simulink model "saturn_thermal5"  (R2021a)
settings: Solver=ode23t  StartTime=0.0  StopTime=t_simul  MaxStep=3600  MinStep=1  RelTol=0.1
values from neighbouring files (symbols this model uses):
  Ab = L*l    [Data_ini_thermal_analysis4.m]    (also in Data_ini_thermal_analysis5.m)
  Ant_Heater_MaxPower = 250    [Data_ini_thermal_analysis5.m]
  As = l*l    [Data_ini_thermal_analysis4.m]    (also in Data_ini_thermal_analysis5.m)
  D_st = 1224526    [Data_ini_thermal_analysis4.m]    (also in Data_ini_thermal_analysis5.m)
  ecc_sc = 0    [Data_ini_thermal_analysis4.m]    (also in Data_ini_thermal_analysis5.m)
  ecc_t = 0.0293    [Data_ini_thermal_analysis4.m]    (also in Data_ini_thermal_analysis5.m)
  Gr_al = sigma*epsilon_al*F_ds    (= 4.3092e-08)    [Data_ini_thermal_analysis4.m]    (also in Data_ini_thermal_analysis5.m)
  incl_ax_s = deg2rad(26.73)    [Data_ini_thermal_analysis4.m]    (also in Data_ini_thermal_analysis5.m)
  incl_sc = deg2rad(90+45)    [Data_ini_thermal_analysis4.m]    (also in Data_ini_thermal_analysis5.m)
  incl_t = deg2rad(0.3485)    [Data_ini_thermal_analysis4.m]    (also in Data_ini_thermal_analysis5.m)
  mean_motion_sc = 2*pi/period_sc    [Data_ini_thermal_analysis4.m]    (also in Data_ini_thermal_analysis5.m)
  mean_motion_t = (2*pi)/period_t    (= 4.56068561416e-06)    [Data_ini_thermal_analysis4.m]    (also in Data_ini_thermal_analysis5.m)
  mean_r_s = 1.427*10^9    (= 1427000000)    [Data_ini_thermal_analysis4.m]    (also in Data_ini_thermal_analysis5.m)
  mu_s = 37931187    [Data_ini_thermal_analysis4.m]    (also in Data_ini_thermal_analysis5.m)
  mu_t = 8971.15    [Data_ini_thermal_analysis4.m]    (also in Data_ini_thermal_analysis5.m)
  period_s = 29.45*365*24*3600    (= 928735200)    [Data_ini_thermal_analysis4.m]    (also in Data_ini_thermal_analysis5.m)
  period_t = 15.945421*24*3600    (= 1377684.3744)    [Data_ini_thermal_analysis4.m]    (also in Data_ini_thermal_analysis5.m)
  R_s = diam_s/2    (= 60268)    [Data_ini_thermal_analysis4.m]    (also in Data_ini_thermal_analysis5.m)
  R_t = 2576    [Data_ini_thermal_analysis4.m]    (also in Data_ini_thermal_analysis5.m)
  rho_al = 0.00277*10^6    (= 2770)    [Data_ini_thermal_analysis4.m]    (also in Data_ini_thermal_analysis5.m)
  semajax_sc = 1500+R_t    (= 4076)    [Data_ini_thermal_analysis4.m]    (also in Data_ini_thermal_analysis5.m)
  semajax_t = 1221830    [Data_ini_thermal_analysis4.m]    (also in Data_ini_thermal_analysis5.m)
  T_ds = 3    [Data_ini_thermal_analysis4.m]    (also in Data_ini_thermal_analysis5.m)
  Vol = 5    [Data_ini_thermal_analysis4.m]    (also in Data_ini_thermal_analysis5.m = 1.3)
libraries: fl_lib x273, nesl_utility x23, pid_lib x2
(part 2 of 3)

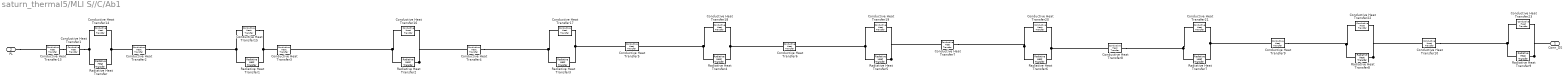
== system saturn_thermal5/MLI S//C/Ab1 ==
  Conductive Heat Transfer{1..10} (10 alike) : fl_lib/Thermal/Thermal Elements/Conductive Heat Transfer  area=Ab m^2  thickness=s_kap m  th_cond=k_kap W/(m*K)  T_specify=off  T_priority=None  T=0 K  T_nominal_specify=off  T_nominal_unit=K  T_nominal_value=1  Q_specify=off  Q_priority=None  Q=0 W  Q_nominal_specify=off  Q_nominal_unit=W  Q_nominal_value=1
  Conductive Heat Transfer13 : fl_lib/Thermal/Thermal Elements/Conductive Heat Transfer  area=Ab m^2  thickness=s_al m  th_cond=k_al W/(m*K)  T_specify=off  T_priority=None  T=0 K  T_nominal_specify=off  T_nominal_unit=K  T_nominal_value=1  Q_specify=off  Q_priority=None  Q=0 W  Q_nominal_specify=off  Q_nominal_unit=W  Q_nominal_value=1
  Conductive Heat Transfer{14..23} (10 alike) : fl_lib/Thermal/Thermal Elements/Conductive Heat Transfer  area=A_net_new_b m^2  thickness=s_tfe_out m  th_cond=k_tfe W/(m*K)  T_specify=off  T_priority=None  T=0 K  T_nominal_specify=off  T_nominal_unit=K  T_nominal_value=1  Q_specify=off  Q_priority=None  Q=0 W  Q_nominal_specify=off  Q_nominal_unit=W  Q_nominal_value=1
  Radiative Heat Transfer{,1..9} (10 alike) : fl_lib/Thermal/Thermal Elements/Radiative Heat Transfer  area=A_empty_b m^2  rad_tr_coeff=Gr_kap_mli W/(m^2*K^4)  T_specify=off  T_priority=None  T=0 K  T_nominal_specify=off  T_nominal_unit=K  T_nominal_value=1  Q_specify=off  Q_priority=None  Q=0 W  Q_nominal_specify=off  Q_nominal_unit=W  Q_nominal_value=1
      settings: SourceProductBaseCode=SS  InternalSimscapePortConfiguration="{\"Bottom\":[],\"Left\":[{\"id\":\"A\",\"label\":\"A\",\"type\":\"foundation.thermal.thermal\"}],\"Right\":[{\"id\":\"B\",\"label\":\"B\",\"type\":\"foundation.thermal.thermal\"}],\"Top\":[]}"
  Conn_DS : PMIOPort  Side=Right
  PL : PMIOPort  Port=2  Side=Left
  connections:
  Conductive Heat Transfer19/LConn1 -- Radiative Heat Transfer5/LConn1 -- Conductive Heat Transfer6/RConn1
  Conductive Heat Transfer20/RConn1 -- Radiative Heat Transfer6/RConn1 -- Conductive Heat Transfer8/LConn1
  Conductive Heat Transfer21/LConn1 -- Radiative Heat Transfer7/LConn1 -- Conductive Heat Transfer8/RConn1
  Conductive Heat Transfer17/LConn1 -- Radiative Heat Transfer3/LConn1 -- Conductive Heat Transfer4/RConn1
  Radiative Heat Transfer5/RConn1 -- Conductive Heat Transfer19/RConn1 -- Conductive Heat Transfer7/LConn1
  Radiative Heat Transfer/LConn1 -- Conductive Heat Transfer1/RConn1 -- Conductive Heat Transfer14/LConn1
  Radiative Heat Transfer4/LConn1 -- Conductive Heat Transfer18/LConn1 -- Conductive Heat Transfer5/RConn1
  Conductive Heat Transfer7/RConn1 -- Conductive Heat Transfer20/LConn1 -- Radiative Heat Transfer6/LConn1
  Conductive Heat Transfer9/LConn1 -- Conductive Heat Transfer21/RConn1 -- Radiative Heat Transfer7/RConn1
  Conductive Heat Transfer18/RConn1 -- Radiative Heat Transfer4/RConn1 -- Conductive Heat Transfer6/LConn1
  Conductive Heat Transfer5/LConn1 -- Conductive Heat Transfer17/RConn1 -- Radiative Heat Transfer3/RConn1
  Radiative Heat Transfer9/LConn1 -- Conductive Heat Transfer23/LConn1 -- Conductive Heat Transfer10/RConn1
  Radiative Heat Transfer/RConn1 -- Conductive Heat Transfer14/RConn1 -- Conductive Heat Transfer2/LConn1
  Radiative Heat Transfer2/LConn1 -- Conductive Heat Transfer16/LConn1 -- Conductive Heat Transfer3/RConn1
  Radiative Heat Transfer2/RConn1 -- Conductive Heat Transfer16/RConn1 -- Conductive Heat Transfer4/LConn1
  Conductive Heat Transfer3/LConn1 -- Conductive Heat Transfer15/RConn1 -- Radiative Heat Transfer1/RConn1
  Radiative Heat Transfer9/RConn1 -- Conductive Heat Transfer23/RConn1 -- Conn_DS/RConn1
  Conductive Heat Transfer15/LConn1 -- Radiative Heat Transfer1/LConn1 -- Conductive Heat Transfer2/RConn1
  Radiative Heat Transfer8/LConn1 -- Conductive Heat Transfer22/LConn1 -- Conductive Heat Transfer9/RConn1
  Radiative Heat Transfer8/RConn1 -- Conductive Heat Transfer22/RConn1 -- Conductive Heat Transfer10/LConn1
  PL/RConn1 -- Conductive Heat Transfer13/LConn1
  Conductive Heat Transfer13/RConn1 -- Conductive Heat Transfer1/LConn1

== system saturn_thermal5/Subsystem/Eclipses System1 ==
  Add : Sum
  Constant : Constant  Value=0
  Saturn-Titan-SC : Subsystem
  Sun-Saturn-Titan : Subsystem
  Sun-Titan-SC : Subsystem
  Out1 : Outport
  ON/OFF : Outport  Port=2
  ON/OFF1 : Outport  Port=3
  ON/OFF2 : Outport  Port=4
  Out5 : Outport  Port=5
  wires:
  Add/1 -> Out1/1
  Sun-Saturn-Titan/1(ON/OFF) -> Add/1, ON/OFF/1
  Saturn-Titan-SC/1(ON/OFF) -> ON/OFF2/1
  Constant/1 -> Out5/1
  Sun-Titan-SC/1(ON/OFF) -> Add/2, ON/OFF1/1

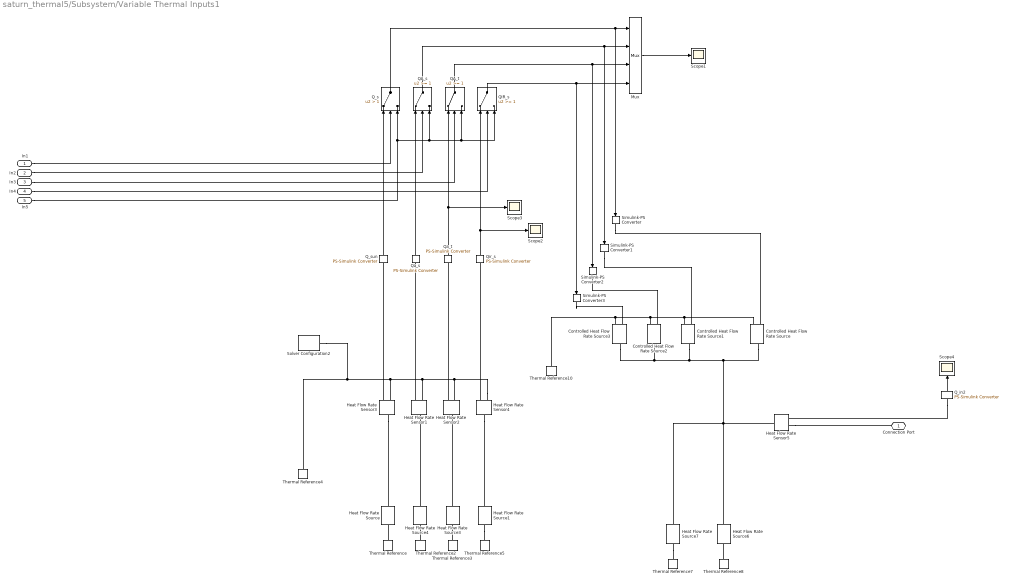
== system saturn_thermal5/Subsystem/Variable Thermal Inputs1 ==
  In1 : Inport
  In2 : Inport  Port=2
  In3 : Inport  Port=3
  In4 : Inport  Port=4
  In5 : Inport  Port=5
  Controlled Heat Flow Rate Source{,1..3} (4 alike) : fl_lib/Thermal/Thermal Sources/Controlled Heat Flow Rate Source
  Heat Flow Rate Sensor{1..5} (5 alike) : fl_lib/Thermal/Thermal Sensors/Heat Flow Rate Sensor
      settings: SourceProductBaseCode=SS
  Heat Flow Rate Source : fl_lib/Thermal/Thermal Sources/Heat Flow Rate Source  heat_flow=Qs_s W
      settings: SourceProductBaseCode=SS  InternalSimscapePortConfiguration="{\"Bottom\":[],\"Left\":[{\"id\":\"B\",\"label\":\"B\",\"type\":\"foundation.thermal.thermal\"}],\"Right\":[{\"id\":\"A\",\"label\":\"A\",\"type\":\"foundation.thermal.thermal\"}],\"Top\":[]}"
  Heat Flow Rate Source1 : fl_lib/Thermal/Thermal Sources/Heat Flow Rate Source  heat_flow=Qir_s W
      settings: SourceProductBaseCode=SS  InternalSimscapePortConfiguration="{\"Bottom\":[],\"Left\":[{\"id\":\"B\",\"label\":\"B\",\"type\":\"foundation.thermal.thermal\"}],\"Right\":[{\"id\":\"A\",\"label\":\"A\",\"type\":\"foundation.thermal.thermal\"}],\"Top\":[]}"
  Heat Flow Rate Source3 : fl_lib/Thermal/Thermal Sources/Heat Flow Rate Source  heat_flow=Qa_t W
      settings: SourceProductBaseCode=SS  InternalSimscapePortConfiguration="{\"Bottom\":[],\"Left\":[{\"id\":\"B\",\"label\":\"B\",\"type\":\"foundation.thermal.thermal\"}],\"Right\":[{\"id\":\"A\",\"label\":\"A\",\"type\":\"foundation.thermal.thermal\"}],\"Top\":[]}"
  Heat Flow Rate Source4 : fl_lib/Thermal/Thermal Sources/Heat Flow Rate Source  heat_flow=Qa_s W
      settings: SourceProductBaseCode=SS  InternalSimscapePortConfiguration="{\"Bottom\":[],\"Left\":[{\"id\":\"B\",\"label\":\"B\",\"type\":\"foundation.thermal.thermal\"}],\"Right\":[{\"id\":\"A\",\"label\":\"A\",\"type\":\"foundation.thermal.thermal\"}],\"Top\":[]}"
  Heat Flow Rate Source6 : fl_lib/Thermal/Thermal Sources/Heat Flow Rate Source  heat_flow=45 W
      settings: SourceProductBaseCode=SS  InternalSimscapePortConfiguration="{\"Bottom\":[],\"Left\":[{\"id\":\"B\",\"label\":\"B\",\"type\":\"foundation.thermal.thermal\"}],\"Right\":[{\"id\":\"A\",\"label\":\"A\",\"type\":\"foundation.thermal.thermal\"}],\"Top\":[]}"
  Heat Flow Rate Source7 : fl_lib/Thermal/Thermal Sources/Heat Flow Rate Source  heat_flow=Qir_t W
      settings: SourceProductBaseCode=SS  InternalSimscapePortConfiguration="{\"Bottom\":[],\"Left\":[{\"id\":\"B\",\"label\":\"B\",\"type\":\"foundation.thermal.thermal\"}],\"Right\":[{\"id\":\"A\",\"label\":\"A\",\"type\":\"foundation.thermal.thermal\"}],\"Top\":[]}"
  Mux : Mux
  QA_s : Switch  Threshold=1
  QA_t : Switch  Threshold=1
  QIR_s : Switch  Threshold=1
  Q_in2 : nesl_utility/PS-Simulink Converter  PhysicalDomain=network_engine_domain  SubClassName=ps_output  LeftPortType=input  RightPortType=output  PseudoPeriodic=off  Frequencies=[]  Unit=inherit  AffineConversion=off
      settings: SourceProductBaseCode=PW,SS
  Q_s : Switch  Criteria=u2 > Threshold  Threshold=1
  Q_sun : nesl_utility/PS-Simulink Converter  PhysicalDomain=network_engine_domain  SubClassName=ps_output  LeftPortType=input  RightPortType=output  PseudoPeriodic=off  Frequencies=[]  Unit=inherit  AffineConversion=off
      settings: SourceProductBaseCode=PW,SS
  Qa_s : nesl_utility/PS-Simulink Converter  PhysicalDomain=network_engine_domain  SubClassName=ps_output  LeftPortType=input  RightPortType=output  PseudoPeriodic=off  Frequencies=[]  Unit=inherit  AffineConversion=off
      settings: SourceProductBaseCode=PW,SS
  Qa_t : nesl_utility/PS-Simulink Converter  PhysicalDomain=network_engine_domain  SubClassName=ps_output  LeftPortType=input  RightPortType=output  PseudoPeriodic=off  Frequencies=[]  Unit=inherit  AffineConversion=off
      settings: SourceProductBaseCode=PW,SS
  Qir_s : nesl_utility/PS-Simulink Converter  PhysicalDomain=network_engine_domain  SubClassName=ps_output  LeftPortType=input  RightPortType=output  PseudoPeriodic=off  Frequencies=[]  Unit=inherit  AffineConversion=off
      settings: SourceProductBaseCode=PW,SS
  Scope{1..4} (4 alike) : Scope
  Simulink-PS Converter{,1..3} (4 alike) : nesl_utility/Simulink-PS Converter  PhysicalDomain=network_engine_domain  SubClassName=ps_input  LeftPortType=input  RightPortType=output  PseudoPeriodic=off  Frequencies=[]  NoiseDistribution=none  NoiseParameters=[]  Unit=1  AffineConversion=off  FilteringAndDerivatives=provide  SimscapeFilterOrder=1  InputFilterTimeConstant=0.001  UdotUserProvided=0
      settings: SourceProductBaseCode=PW,SS
  Solver Configuration2 : nesl_utility/Solver Configuration  PhysicalDomain=network_engine_domain  SubClassName=solver  LeftPortType=input  RightPortType=generic  Tones=[]  Harmonics=[]  SimulateNoise=off  Profile=off  UseLocalSampling=off  EnableSwitchedLinearOptims=on  FrequencyDomain=off  UseCCode=off  RelTol=0.001  AbsTol=1e-06  MinStep=1e-09  ToWorkspace=off  RevertToSquareIcSolve=off  NumHomotopyIterations=100  PhasorMode=off  PhasorModeNumHarmonics=1  DoDC=off  ResidualTolerance=1e-09  UseLocalSolver=off  LocalSolverChoice=NE_BACKWARD_EULER_ADVANCER  LocalSolverSampleTime=0.001  DoFixedCost=off  MaxNonlinIter=3  MaxModeIter=2  ComputeImpulses=off  ImpulseIterations=2  LinearAlgebra=auto  EquationFormulation=NE_TIME_EF  DelaysMemoryBudget=1024  AutomaticFiltering=on  FilteringTimeConstant=0.001  PartitionStorageMethod=AS_NEEDED  PartitionMemoryBudget=1024  PartitionMethod=ROBUST
      settings: SourceProductBaseCode=PW,SS
  Thermal Reference{,2..5,7..8,10} (8 alike) : fl_lib/Thermal/Thermal Elements/Thermal Reference
  Connection Port : PMIOPort  Side=Right
  wires:
  Q_in2/1 -> Scope4/1
  In3/1 -> QA_t/2
  In1/1 -> Q_s/2
  In2/1 -> QA_s/2
  In4/1 -> QIR_s/2
  Mux/1 -> Scope1/1
  Qir_s/1 -> Scope2/1, QIR_s/1
  Q_s/1 -> Mux/1, Simulink-PS Converter/1
  Q_sun/1 -> Q_s/1
  Qa_t/1 -> QA_t/1, Scope3/1
  QA_s/1 -> Mux/2, Simulink-PS Converter1/1
  QIR_s/1 -> Mux/4, Simulink-PS Converter3/1
  Qa_s/1 -> QA_s/1
  In5/1 -> Q_s/3, QA_t/3, QIR_s/3, QA_s/3
  QA_t/1 -> Mux/3, Simulink-PS Converter2/1
  connections:
  Heat Flow Rate Sensor5/RConn2 -- Connection Port/RConn1
  Controlled Heat Flow Rate Source1/LConn1 -- Controlled Heat Flow Rate Source2/LConn1 -- Controlled Heat Flow Rate Source3/LConn1 -- Controlled Heat Flow Rate Source/LConn1 -- Heat Flow Rate Source7/LConn1 -- Heat Flow Rate Sensor5/LConn1 -- Heat Flow Rate Source6/LConn1
  Q_in2/LConn1 -- Heat Flow Rate Sensor5/RConn1
  Heat Flow Rate Sensor3/LConn1 -- Heat Flow Rate Source/LConn1
  Heat Flow Rate Sensor2/LConn1 -- Heat Flow Rate Source3/LConn1
  Heat Flow Rate Sensor4/LConn1 -- Heat Flow Rate Source1/LConn1
  Heat Flow Rate Sensor3/RConn1 -- Q_sun/LConn1
  Simulink-PS Converter/RConn1 -- Controlled Heat Flow Rate Source/RConn1
  Heat Flow Rate Source7/RConn1 -- Thermal Reference7/LConn1
  Heat Flow Rate Sensor4/RConn1 -- Qir_s/LConn1
  Heat Flow Rate Sensor1/RConn1 -- Qa_s/LConn1
  Simulink-PS Converter3/RConn1 -- Controlled Heat Flow Rate Source3/RConn1
  Simulink-PS Converter2/RConn1 -- Controlled Heat Flow Rate Source2/RConn1
  Simulink-PS Converter1/RConn1 -- Controlled Heat Flow Rate Source1/RConn1
  Thermal Reference/LConn1 -- Heat Flow Rate Source/RConn1
  Heat Flow Rate Sensor2/RConn1 -- Qa_t/LConn1
  Heat Flow Rate Source1/RConn1 -- Thermal Reference5/LConn1
  Thermal Reference3/LConn1 -- Heat Flow Rate Source3/RConn1
  Controlled Heat Flow Rate Source2/RConn2 -- Controlled Heat Flow Rate Source1/RConn2 -- Controlled Heat Flow Rate Source/RConn2 -- Controlled Heat Flow Rate Source3/RConn2 -- Thermal Reference10/LConn1
  Heat Flow Rate Source4/RConn1 -- Thermal Reference2/LConn1
  Heat Flow Rate Sensor1/LConn1 -- Heat Flow Rate Source4/LConn1
  Thermal Reference8/LConn1 -- Heat Flow Rate Source6/RConn1
  Heat Flow Rate Sensor4/RConn2 -- Heat Flow Rate Sensor2/RConn2 -- Heat Flow Rate Sensor1/RConn2 -- Heat Flow Rate Sensor3/RConn2 -- Solver Configuration2/RConn1 -- Thermal Reference4/LConn1

== system saturn_thermal5/active heat control box/Subsystem ==
  signal : Inport
  temp_goal : Inport  Port=2
  Controlled Heat Flow Rate Source : fl_lib/Thermal/Thermal Sources/Controlled Heat Flow Rate Source
  Data Type Conversion : DataTypeConversion  OutDataTypeStr=double
  Data Type Conversion1 : DataTypeConversion  OutDataTypeStr=boolean
  Scope : Scope
  Simulink-PS Converter : nesl_utility/Simulink-PS Converter  PhysicalDomain=network_engine_domain  SubClassName=ps_input  LeftPortType=input  RightPortType=output  PseudoPeriodic=off  Frequencies=[]  NoiseDistribution=none  NoiseParameters=[]  Unit=1  AffineConversion=off  FilteringAndDerivatives=provide  SimscapeFilterOrder=1  InputFilterTimeConstant=0.001  UdotUserProvided=0
      settings: SourceProductBaseCode=PW,SS
  Subsystem : Subsystem
  Subtract : Sum  Inputs=-+
  Thermal Reference1 : fl_lib/Thermal/Thermal Elements/Thermal Reference
  heat block : PMIOPort  Side=Right
  Output : Outport
  wires:
  Data Type Conversion/1 -> Simulink-PS Converter/1
  Subtract/1 -> Subsystem/1(Error)
  signal/1 -> Subtract/1
  temp_goal/1 -> Subtract/2
  Subsystem/1(Output) -> Data Type Conversion1/1, Scope/1, Data Type Conversion/1
  Data Type Conversion1/1 -> Output/1
  connections:
  Thermal Reference1/LConn1 -- Controlled Heat Flow Rate Source/RConn2
  Controlled Heat Flow Rate Source/LConn1 -- heat block/RConn1
  Simulink-PS Converter/RConn1 -- Controlled Heat Flow Rate Source/RConn1

== system saturn_thermal5/active heat control box/Subsystem1 ==
  signal : Inport
  reference : Inport  Port=2
  Controlled Temperature Source : fl_lib/Thermal/Thermal Sources/Controlled Temperature Source
  Gain : Gain  Gain=T_ds
  PS-Simulink Converter : nesl_utility/PS-Simulink Converter  PhysicalDomain=network_engine_domain  SubClassName=ps_output  LeftPortType=input  RightPortType=output  PseudoPeriodic=off  Frequencies=[]  Unit=inherit  AffineConversion=off
      settings: SourceProductBaseCode=PW,SS
  Product : Product
  Radiative Heat Transfer : fl_lib/Thermal/Thermal Elements/Radiative Heat Transfer  area=Ab m^2  rad_tr_coeff=Gr_cu W/(m^2*K^4)  T_specify=off  T_priority=None  T=0 K  T_nominal_specify=off  T_nominal_unit=K  T_nominal_value=1  Q_specify=off  Q_priority=None  Q=0 W  Q_nominal_specify=off  Q_nominal_unit=W  Q_nominal_value=1
      settings: SourceProductBaseCode=SS  InternalSimscapePortConfiguration="{\"Bottom\":[],\"Left\":[{\"id\":\"A\",\"label\":\"A\",\"type\":\"foundation.thermal.thermal\"}],\"Right\":[{\"id\":\"B\",\"label\":\"B\",\"type\":\"foundation.thermal.thermal\"}],\"Top\":[]}"
  Relational Operator : RelationalOperator  Operator=>  OutDataTypeStr=boolean  RndMeth=Simplest
  Relational Operator1 : RelationalOperator  Operator=<=  OutDataTypeStr=boolean  RndMeth=Simplest
  Simulink-PS Converter : nesl_utility/Simulink-PS Converter  PhysicalDomain=network_engine_domain  SubClassName=ps_input  LeftPortType=input  RightPortType=output  PseudoPeriodic=off  Frequencies=[]  NoiseDistribution=none  NoiseParameters=[]  Unit=1  AffineConversion=off  FilteringAndDerivatives=zero  SimscapeFilterOrder=1  InputFilterTimeConstant=0.001  UdotUserProvided=0
      settings: SourceProductBaseCode=PW,SS
  Sum : Sum  Inputs=|++
  Temperature Sensor : fl_lib/Thermal/Thermal Sensors/Temperature Sensor
  Thermal Reference : fl_lib/Thermal/Thermal Elements/Thermal Reference
  heat block : PMIOPort  Side=Left
  Output : Outport
  wires:
  signal/1 -> Relational Operator1/1, Relational Operator/1
  reference/1 -> Relational Operator1/2, Relational Operator/2
  Relational Operator/1 -> Output/1, Gain/1
  Relational Operator1/1 -> Product/2
  PS-Simulink Converter/1 -> Product/1
  Product/1 -> Sum/1
  Gain/1 -> Sum/2
  Sum/1 -> Simulink-PS Converter/1
  connections:
  Temperature Sensor/RConn1 -- Thermal Reference/LConn1 -- Controlled Temperature Source/RConn2
  Simulink-PS Converter/RConn1 -- Controlled Temperature Source/RConn1
  PS-Simulink Converter/LConn1 -- Temperature Sensor/RConn2
  Radiative Heat Transfer/LConn1 -- Temperature Sensor/LConn1 -- heat block/RConn1
  Controlled Temperature Source/LConn1 -- Radiative Heat Transfer/RConn1

== system saturn_thermal5/active heat control ref + antenna/Subsystem ==
  signal : Inport
  temp_goal : Inport  Port=2
  Controlled Heat Flow Rate Source : fl_lib/Thermal/Thermal Sources/Controlled Heat Flow Rate Source
  Data Type Conversion : DataTypeConversion  OutDataTypeStr=double
  Data Type Conversion1 : DataTypeConversion  OutDataTypeStr=boolean
  Scope : Scope
  Simulink-PS Converter : nesl_utility/Simulink-PS Converter  PhysicalDomain=network_engine_domain  SubClassName=ps_input  LeftPortType=input  RightPortType=output  PseudoPeriodic=off  Frequencies=[]  NoiseDistribution=none  NoiseParameters=[]  Unit=1  AffineConversion=off  FilteringAndDerivatives=provide  SimscapeFilterOrder=1  InputFilterTimeConstant=0.001  UdotUserProvided=0
      settings: SourceProductBaseCode=PW,SS
  Subsystem : Subsystem
  Subtract : Sum  Inputs=-+
  Thermal Reference1 : fl_lib/Thermal/Thermal Elements/Thermal Reference
  heat block : PMIOPort  Side=Right
  Output : Outport
  wires:
  Data Type Conversion/1 -> Simulink-PS Converter/1
  Subtract/1 -> Subsystem/1(Error)
  signal/1 -> Subtract/1
  temp_goal/1 -> Subtract/2
  Subsystem/1(Output) -> Data Type Conversion1/1, Scope/1, Data Type Conversion/1
  Data Type Conversion1/1 -> Output/1
  connections:
  Thermal Reference1/LConn1 -- Controlled Heat Flow Rate Source/RConn2
  Controlled Heat Flow Rate Source/LConn1 -- heat block/RConn1
  Simulink-PS Converter/RConn1 -- Controlled Heat Flow Rate Source/RConn1

== system saturn_thermal5/Subsystem/Eclipses System1/Saturn-Titan-SC ==
  S/C Titan Saturn : Subsystem
  S/C-Titan orbit : Subsystem
  Titan-Saturn orbit : Subsystem
  ON/OFF : Outport
  wires:
  S/C Titan Saturn/1(ON/OFF) -> ON/OFF/1
  Titan-Saturn orbit/1(S_mn) -> S/C Titan Saturn/1(S_mn)
  S/C-Titan orbit/1(r_mn) -> S/C Titan Saturn/2(r_mn)

== system saturn_thermal5/Subsystem/Eclipses System1/Sun-Saturn-Titan ==
  Saturn-Sun orbit : Subsystem
  Titan-Saturn : Subsystem
  Titan-Saturn-Sun Eclipse : Subsystem
  ON/OFF : Outport
  wires:
  Titan-Saturn-Sun Eclipse/1(ON/OFF) -> ON/OFF/1
  Titan-Saturn/1(r_mn) -> Titan-Saturn-Sun Eclipse/2(r_mn)
  Saturn-Sun orbit/1(S_mn) -> Titan-Saturn-Sun Eclipse/1(S_mn)

== system saturn_thermal5/Subsystem/Eclipses System1/Sun-Titan-SC ==
  Ecliptic Orbital parameter1 : Subsystem
  Orbit Parameter1 : Subsystem
  S/C Titan Sun Eclipse : Subsystem
  ON/OFF : Outport
  wires:
  S/C Titan Sun Eclipse/1(ON/OFF) -> ON/OFF/1
  Orbit Parameter1/1(r_mn) -> S/C Titan Sun Eclipse/2(r_mn)
  Ecliptic Orbital parameter1/1(S_mn) -> S/C Titan Sun Eclipse/1(S_mn)

== system saturn_thermal5/active heat control box/Subsystem/Subsystem ==
  Error : Inport
  PID Controller : pid_lib/PID Controller  Controller=PID  Form=Parallel  TimeDomain=Continuous-time  UseExternalTs=off  SampleTime=-1  IntegratorMethod=Forward Euler  FilterMethod=Forward Euler  ControllerParametersSource=internal  P=0.05  I=0.005  D=0.01  UseFilter=on  N=1  TunerSelectOption=Frequency Response Based  InitialConditionSource=internal  InitialConditionForIntegrator=0  InitialConditionForFilter=0  DifferentiatorICPrevScaledInput=0  ExternalReset=none  TrackingMode=off  Kt=1  LimitOutput=off  SatLimitsSource=internal  UpperSaturationLimit=inf  LowerSaturationLimit=-inf  LinearizeAsGain=on  AntiWindupMode=none  Kb=1  POutMin=[]  POutMax=[]  IOutMin=[]  IOutMax=[]  DOutMin=[]  DOutMax=[]  NOutMin=[]  NOutMax=[]  SumOutMin=[]  SumOutMax=[]  SaturationOutMin=[]  SaturationOutMax=[]  PParamMin=[]  PParamMax=[]  IParamMin=[]  IParamMax=[]  DParamMin=[]  DParamMax=[]  NParamMin=[]  NParamMax=[]  KbParamMin=[]  KbParamMax=[]  KtParamMin=[]  KtParamMax=[]  KbOutMin=[]  KbOutMax=[]  KtOutMin=[]  KtOutMax=[]  IntegratorOutMin=[]  IntegratorOutMax=[]  FilterOutMin=[]  FilterOutMax=[]  SumI1OutMin=[]  SumI1OutMax=[]  SumI2OutMin=[]  SumI2OutMax=[]  SumI3OutMin=[]  SumI3OutMax=[]  SumI4OutMin=[]  SumI4OutMax=[]  SumDOutMin=[]  SumDOutMax=[]  DifferentiatorOutMin=[]  DifferentiatorOutMax=[]  FilterDiffOutCoefMin=[]  FilterDiffOutCoefMax=[]  ReciprocalOutMin=[]  ReciprocalOutMax=[]  SumDenOutMin=[]  SumDenOutMax=[]  SumNumOutMin=[]  SumNumOutMax=[]  DivideOutMin=[]  DivideOutMax=[]  UdiffTsProdOutMin=[]  UdiffTsProdOutMax=[]  NTsProdOutMin=[]  NTsProdOutMax=[]  UintegralTsProdOutMin=[]  UintegralTsProdOutMax=[]  UngainTsProdOutMin=[]  UngainTsProdOutMax=[]  IntegratorContinuousStateAttributes=''  IntegratorStateMustResolveToSignalObject=off  IntegratorRTWStateStorageClass=Auto  FilterContinuousStateAttributes=''  FilterStateMustResolveToSignalObject=off  FilterRTWStateStorageClass=Auto  ParallelPVariant=InternalParameters  IdealPVariant=Disabled  IVariant=InternalParameters  DVariant=InternalParameters  IntegratorVariant=Continuous  SatVariant=Disabled  AWVariant=Passthrough  PCopyVariant=Disabled  TRVariant=Disabled  FdbkBlocksVariant=Forward  IdealPFdbkVariant=Disabled  SatFdbkVariant=Disabled  DerivativeFilterVariant=ContFilter  NVariant=InternalParameters  NCopyVariant=Disabled  FilterICVariant=InternalICsFilter  IntegratorICVariant=InternalICs  ExternalResetVariant=Disabled  TRSumVariant=Passthrough  SumFdbkVariant=Disabled  SumVariant=Sum_PID  TsampFilterVariant=InternalTs  TsampNgainVariant=Passthrough  TsampIntegralVariant=Passthrough  ExternalSaturationOutDataTypeStr=Inherit: Same as second input
  Saturation : Saturate  UpperLimit=Ant_Heater_MaxPower-50  LowerLimit=0
  Scope : Scope
  Scope1 : Scope
  Output : Outport
  wires:
  PID Controller/1 -> Saturation/1
  Saturation/1 -> Scope/1, Output/1
  Error/1 -> PID Controller/1, Scope1/1

== system saturn_thermal5/active heat control ref + antenna/Subsystem/Subsystem ==
  Error : Inport
  PID Controller : pid_lib/PID Controller  Controller=PID  Form=Parallel  TimeDomain=Continuous-time  UseExternalTs=off  SampleTime=-1  IntegratorMethod=Forward Euler  FilterMethod=Forward Euler  ControllerParametersSource=internal  P=0.05  I=0.005  D=0.01  UseFilter=on  N=1  TunerSelectOption=Frequency Response Based  InitialConditionSource=internal  InitialConditionForIntegrator=0  InitialConditionForFilter=0  DifferentiatorICPrevScaledInput=0  ExternalReset=none  TrackingMode=off  Kt=1  LimitOutput=off  SatLimitsSource=internal  UpperSaturationLimit=inf  LowerSaturationLimit=-inf  LinearizeAsGain=on  AntiWindupMode=none  Kb=1  POutMin=[]  POutMax=[]  IOutMin=[]  IOutMax=[]  DOutMin=[]  DOutMax=[]  NOutMin=[]  NOutMax=[]  SumOutMin=[]  SumOutMax=[]  SaturationOutMin=[]  SaturationOutMax=[]  PParamMin=[]  PParamMax=[]  IParamMin=[]  IParamMax=[]  DParamMin=[]  DParamMax=[]  NParamMin=[]  NParamMax=[]  KbParamMin=[]  KbParamMax=[]  KtParamMin=[]  KtParamMax=[]  KbOutMin=[]  KbOutMax=[]  KtOutMin=[]  KtOutMax=[]  IntegratorOutMin=[]  IntegratorOutMax=[]  FilterOutMin=[]  FilterOutMax=[]  SumI1OutMin=[]  SumI1OutMax=[]  SumI2OutMin=[]  SumI2OutMax=[]  SumI3OutMin=[]  SumI3OutMax=[]  SumI4OutMin=[]  SumI4OutMax=[]  SumDOutMin=[]  SumDOutMax=[]  DifferentiatorOutMin=[]  DifferentiatorOutMax=[]  FilterDiffOutCoefMin=[]  FilterDiffOutCoefMax=[]  ReciprocalOutMin=[]  ReciprocalOutMax=[]  SumDenOutMin=[]  SumDenOutMax=[]  SumNumOutMin=[]  SumNumOutMax=[]  DivideOutMin=[]  DivideOutMax=[]  UdiffTsProdOutMin=[]  UdiffTsProdOutMax=[]  NTsProdOutMin=[]  NTsProdOutMax=[]  UintegralTsProdOutMin=[]  UintegralTsProdOutMax=[]  UngainTsProdOutMin=[]  UngainTsProdOutMax=[]  IntegratorContinuousStateAttributes=''  IntegratorStateMustResolveToSignalObject=off  IntegratorRTWStateStorageClass=Auto  FilterContinuousStateAttributes=''  FilterStateMustResolveToSignalObject=off  FilterRTWStateStorageClass=Auto  ParallelPVariant=InternalParameters  IdealPVariant=Disabled  IVariant=InternalParameters  DVariant=InternalParameters  IntegratorVariant=Continuous  SatVariant=Disabled  AWVariant=Passthrough  PCopyVariant=Disabled  TRVariant=Disabled  FdbkBlocksVariant=Forward  IdealPFdbkVariant=Disabled  SatFdbkVariant=Disabled  DerivativeFilterVariant=ContFilter  NVariant=InternalParameters  NCopyVariant=Disabled  FilterICVariant=InternalICsFilter  IntegratorICVariant=InternalICs  ExternalResetVariant=Disabled  TRSumVariant=Passthrough  SumFdbkVariant=Disabled  SumVariant=Sum_PID  TsampFilterVariant=InternalTs  TsampNgainVariant=Passthrough  TsampIntegralVariant=Passthrough  ExternalSaturationOutDataTypeStr=Inherit: Same as second input
  Saturation : Saturate  UpperLimit=Ant_Heater_MaxPower-50  LowerLimit=0
  Scope : Scope
  Scope1 : Scope
  Output : Outport
  wires:
  PID Controller/1 -> Saturation/1
  Saturation/1 -> Scope/1, Output/1
  Error/1 -> PID Controller/1, Scope1/1

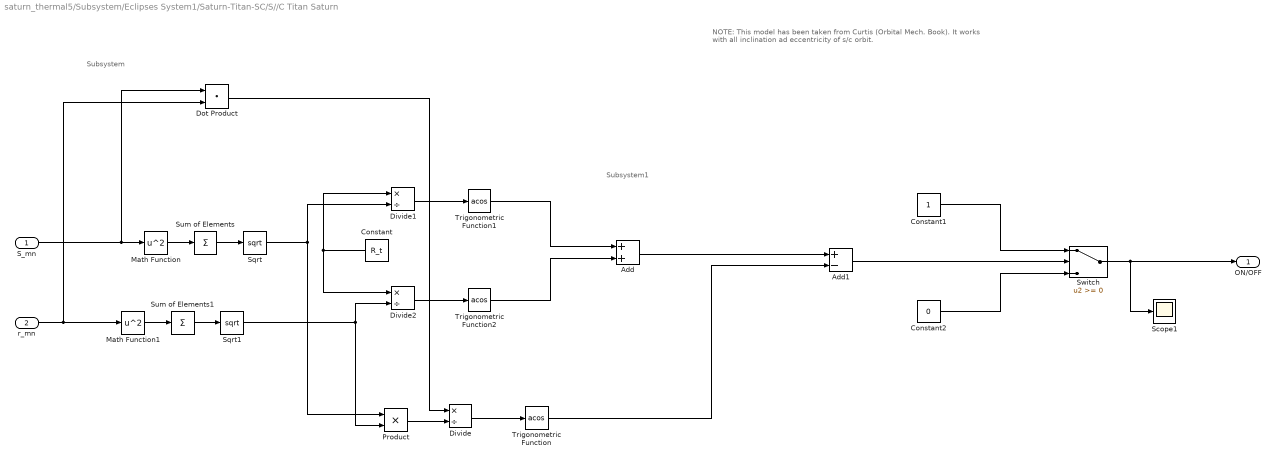
== system saturn_thermal5/Subsystem/Eclipses System1/Saturn-Titan-SC/S//C Titan Saturn ==
  note: NOTE: This model has been taken from Curtis (Orbital Mech. Book). It works with all inclination ad eccentricity of s/c orbit.
  note: Subsystem1
  note: Subsystem
  S_mn : Inport
  r_mn : Inport  Port=2
  Add : Sum
  Add1 : Sum  Inputs=+-
  Constant : Constant  Value=R_t
  Constant1 : Constant
  Constant2 : Constant  Value=0
  Divide : Product  Inputs=*/
  Divide1 : Product  Inputs=*/
  Divide2 : Product  Inputs=*/
  Dot Product : DotProduct  InputSameDT=on  OutDataTypeStr=Inherit: Inherit via internal rule
  Math Function : Math  Operator=square  SaturateOnIntegerOverflow=on
  Math Function1 : Math  Operator=square  SaturateOnIntegerOverflow=on
  Product : Product
  Scope1 : Scope
  Sqrt : Sqrt  SaturateOnIntegerOverflow=on
  Sqrt1 : Sqrt  SaturateOnIntegerOverflow=on
  Sum of Elements : Sum  Inputs=+
  Sum of Elements1 : Sum  Inputs=+
  Switch : Switch
  Trigonometric Function : Trigonometry  Operator=acos
  Trigonometric Function1 : Trigonometry  Operator=acos
  Trigonometric Function2 : Trigonometry  Operator=acos
  ON/OFF : Outport
  wires:
  Switch/1 -> Scope1/1, ON/OFF/1
  Sum of Elements/1 -> Sqrt/1
  Math Function/1 -> Sum of Elements/1
  Divide1/1 -> Trigonometric Function1/1
  Math Function1/1 -> Sum of Elements1/1
  r_mn/1 -> Dot Product/2, Math Function1/1
  Dot Product/1 -> Divide/1
  Divide2/1 -> Trigonometric Function2/1
  Sqrt/1 -> Product/1, Divide1/2
  Product/1 -> Divide/2
  Sqrt1/1 -> Product/2, Divide2/2
  S_mn/1 -> Math Function/1, Dot Product/1
  Constant/1 -> Divide1/1, Divide2/1
  Sum of Elements1/1 -> Sqrt1/1
  Divide/1 -> Trigonometric Function/1
  Trigonometric Function/1 -> Add1/2
  Trigonometric Function2/1 -> Add/2
  Trigonometric Function1/1 -> Add/1
  Constant2/1 -> Switch/3
  Constant1/1 -> Switch/1
  Add1/1 -> Switch/2
  Add/1 -> Add1/1

== system saturn_thermal5/Subsystem/Eclipses System1/Saturn-Titan-SC/S//C-Titan orbit ==
  Inertial Orbit Direction (Theta) : Subsystem
  Inertial Orbit Radius(Theta) : Subsystem
  Product : Product
  Subsystem : Subsystem
  True anomaly integration : Subsystem
  r_mn Scope : Scope
  r_mn : Outport
  wires:
  True anomaly integration/1(Theta) -> Inertial Orbit Radius(Theta)/1(Theta), Inertial Orbit Direction (Theta)/1(Theta)  "Theta"
  Inertial Orbit Radius(Theta)/1(r_mn) -> Product/1, Subsystem/1(r_mn)
  Inertial Orbit Direction (Theta)/1(r_vn) -> Product/2
  Product/1 -> r_mn/1, r_mn Scope/1  "r_mn"

== system saturn_thermal5/Subsystem/Eclipses System1/Saturn-Titan-SC/Titan-Saturn orbit ==
  Constant : Constant  Value=0
  Constant1 : Constant  Value=D_st
  Interpreted MATLAB Function : MATLABFcn  MATLABFcn=norm(u)
  Mux : Mux  Inputs=3
  Product : Product
  Product1 : Product
  Product2 : Product
  Scope : Scope
  Scope1 : Scope
  Subsystem : Subsystem
  Trigonometric Function : Trigonometry
  Trigonometric Function1 : Trigonometry  Operator=cos
  Trigonometric Function2 : Trigonometry
  Trigonometric Function3 : Trigonometry  Operator=cos
  Trigonometric Function4 : Trigonometry
  S_mn : Outport
  wires:
  Product1/1 -> Mux/3
  Trigonometric Function1/1 -> Mux/1
  Constant/1 -> Trigonometric Function4/1, Trigonometric Function3/1
  Subsystem/1(theta_titan) -> Trigonometric Function1/1, Trigonometric Function/1, Trigonometric Function2/1
  Trigonometric Function/1 -> Product/1
  Trigonometric Function4/1 -> Product1/1
  Product/1 -> Mux/2
  Trigonometric Function2/1 -> Product1/2
  Trigonometric Function3/1 -> Product/2
  Constant1/1 -> Product2/1
  Mux/1 -> Interpreted MATLAB Function/1, Product2/2
  Product2/1 -> S_mn/1, Scope/1
  Interpreted MATLAB Function/1 -> Scope1/1

== system saturn_thermal5/Subsystem/Eclipses System1/Sun-Saturn-Titan/Saturn-Sun orbit ==
  Constant : Constant  Value=incl_ax_s
  Constant1 : Constant  Value=mean_r_s
  Interpreted MATLAB Function : MATLABFcn  MATLABFcn=norm(u)
  Mux : Mux  Inputs=3
  Product : Product
  Product1 : Product
  Product2 : Product
  Scope : Scope
  Scope1 : Scope
  Subsystem : Subsystem
  Trigonometric Function : Trigonometry
  Trigonometric Function1 : Trigonometry  Operator=cos
  Trigonometric Function2 : Trigonometry
  Trigonometric Function3 : Trigonometry  Operator=cos
  Trigonometric Function4 : Trigonometry
  S_mn : Outport
  wires:
  Interpreted MATLAB Function/1 -> Scope1/1
  Product2/1 -> Scope/1, S_mn/1
  Mux/1 -> Product2/2, Interpreted MATLAB Function/1
  Constant1/1 -> Product2/1
  Trigonometric Function3/1 -> Product/2
  Trigonometric Function2/1 -> Product1/2
  Product/1 -> Mux/2
  Trigonometric Function4/1 -> Product1/1
  Trigonometric Function/1 -> Product/1
  Subsystem/1(theta_saturn) -> Trigonometric Function2/1, Trigonometric Function/1, Trigonometric Function1/1
  Constant/1 -> Trigonometric Function3/1, Trigonometric Function4/1
  Trigonometric Function1/1 -> Mux/1
  Product1/1 -> Mux/3

== system saturn_thermal5/Subsystem/Eclipses System1/Sun-Saturn-Titan/Titan-Saturn ==
  Inertial Orbit Direction (Theta) : Subsystem
  Inertial Orbit Radius(Theta) : Subsystem
  Product : Product
  Subsystem : Subsystem
  True anomaly integration : Subsystem
  r_mn Scope : Scope
  r_mn : Outport
  wires:
  Product/1 -> r_mn Scope/1, r_mn/1  "r_mn"
  Inertial Orbit Direction (Theta)/1(r_vn) -> Product/2
  Inertial Orbit Radius(Theta)/1(r_mn) -> Subsystem/1(r_mn), Product/1
  True anomaly integration/1(Theta) -> Inertial Orbit Direction (Theta)/1(Theta), Inertial Orbit Radius(Theta)/1(Theta)  "Theta"

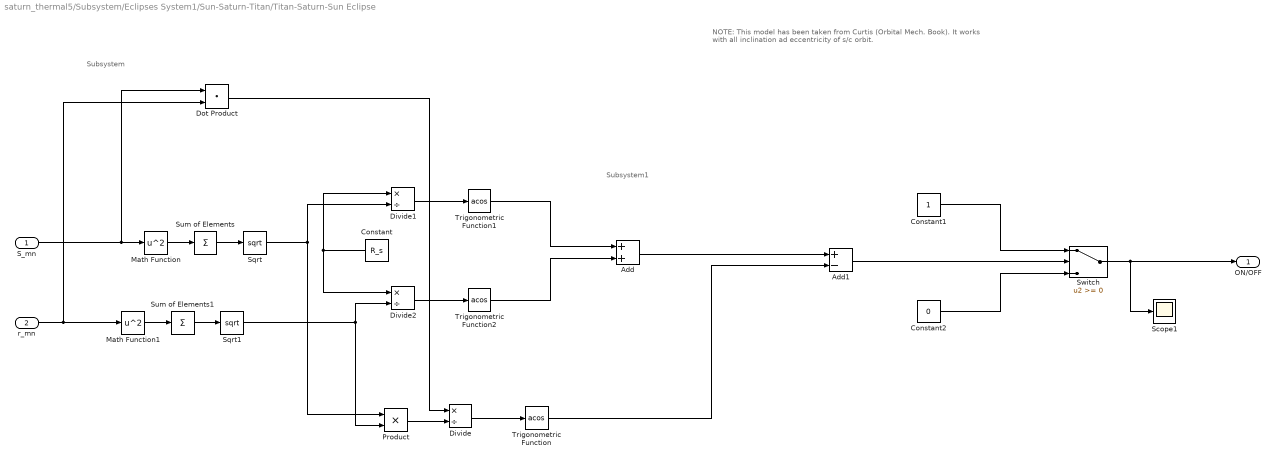
== system saturn_thermal5/Subsystem/Eclipses System1/Sun-Saturn-Titan/Titan-Saturn-Sun Eclipse ==
  note: Subsystem
  note: Subsystem1
  note: NOTE: This model has been taken from Curtis (Orbital Mech. Book). It works with all inclination ad eccentricity of s/c orbit.
  S_mn : Inport
  r_mn : Inport  Port=2
  Add : Sum
  Add1 : Sum  Inputs=+-
  Constant : Constant  Value=R_s
  Constant1 : Constant
  Constant2 : Constant  Value=0
  Divide : Product  Inputs=*/
  Divide1 : Product  Inputs=*/
  Divide2 : Product  Inputs=*/
  Dot Product : DotProduct  InputSameDT=on  OutDataTypeStr=Inherit: Inherit via internal rule
  Math Function : Math  Operator=square  SaturateOnIntegerOverflow=on
  Math Function1 : Math  Operator=square  SaturateOnIntegerOverflow=on
  Product : Product
  Scope1 : Scope
  Sqrt : Sqrt  SaturateOnIntegerOverflow=on
  Sqrt1 : Sqrt  SaturateOnIntegerOverflow=on
  Sum of Elements : Sum  Inputs=+
  Sum of Elements1 : Sum  Inputs=+
  Switch : Switch
  Trigonometric Function : Trigonometry  Operator=acos
  Trigonometric Function1 : Trigonometry  Operator=acos
  Trigonometric Function2 : Trigonometry  Operator=acos
  ON/OFF : Outport
  wires:
  Add/1 -> Add1/1
  Add1/1 -> Switch/2
  Constant1/1 -> Switch/1
  Constant2/1 -> Switch/3
  Trigonometric Function1/1 -> Add/1
  Trigonometric Function2/1 -> Add/2
  Trigonometric Function/1 -> Add1/2
  Divide/1 -> Trigonometric Function/1
  Sum of Elements1/1 -> Sqrt1/1
  Constant/1 -> Divide2/1, Divide1/1
  S_mn/1 -> Dot Product/1, Math Function/1
  Sqrt1/1 -> Divide2/2, Product/2
  Product/1 -> Divide/2
  Sqrt/1 -> Divide1/2, Product/1
  Divide2/1 -> Trigonometric Function2/1
  Dot Product/1 -> Divide/1
  r_mn/1 -> Math Function1/1, Dot Product/2
  Math Function1/1 -> Sum of Elements1/1
  Divide1/1 -> Trigonometric Function1/1
  Math Function/1 -> Sum of Elements/1
  Sum of Elements/1 -> Sqrt/1
  Switch/1 -> ON/OFF/1, Scope1/1

== system saturn_thermal5/Subsystem/Eclipses System1/Sun-Titan-SC/Ecliptic Orbital parameter1 ==
  Constant : Constant  Value=0
  Constant1 : Constant  Value=mean_r_s
  Interpreted MATLAB Function : MATLABFcn  MATLABFcn=norm(u)
  Mux : Mux  Inputs=3
  Product : Product
  Product1 : Product
  Product2 : Product
  Scope : Scope
  Scope1 : Scope
  Subsystem : Subsystem
  Trigonometric Function : Trigonometry
  Trigonometric Function1 : Trigonometry  Operator=cos
  Trigonometric Function2 : Trigonometry
  Trigonometric Function3 : Trigonometry  Operator=cos
  Trigonometric Function4 : Trigonometry
  S_mn : Outport
  wires:
  Product1/1 -> Mux/3
  Trigonometric Function1/1 -> Mux/1
  Constant/1 -> Trigonometric Function4/1, Trigonometric Function3/1
  Subsystem/1(theta_sun) -> Trigonometric Function1/1, Trigonometric Function/1, Trigonometric Function2/1
  Trigonometric Function/1 -> Product/1
  Trigonometric Function4/1 -> Product1/1
  Product/1 -> Mux/2
  Trigonometric Function2/1 -> Product1/2
  Trigonometric Function3/1 -> Product/2
  Constant1/1 -> Product2/1
  Mux/1 -> Interpreted MATLAB Function/1, Product2/2
  Product2/1 -> S_mn/1, Scope/1
  Interpreted MATLAB Function/1 -> Scope1/1

== system saturn_thermal5/Subsystem/Eclipses System1/Sun-Titan-SC/Orbit Parameter1 ==
  Inertial Orbit Direction (Theta) : Subsystem
  Inertial Orbit Radius(Theta) : Subsystem
  Product : Product
  Subsystem : Subsystem
  True anomaly integration : Subsystem
  r_mn Scope : Scope
  r_mn : Outport
  wires:
  True anomaly integration/1(Theta) -> Inertial Orbit Radius(Theta)/1(Theta), Inertial Orbit Direction (Theta)/1(Theta)  "Theta"
  Inertial Orbit Radius(Theta)/1(r_mn) -> Product/1, Subsystem/1(r_mn)
  Inertial Orbit Direction (Theta)/1(r_vn) -> Product/2
  Product/1 -> r_mn/1, r_mn Scope/1  "r_mn"

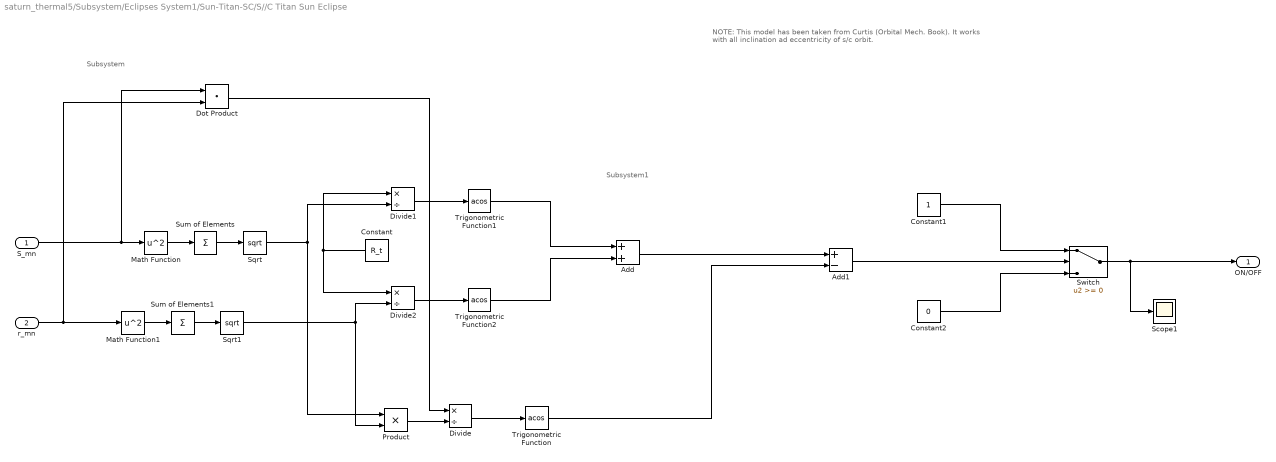
== system saturn_thermal5/Subsystem/Eclipses System1/Sun-Titan-SC/S//C Titan Sun Eclipse ==
  note: NOTE: This model has been taken from Curtis (Orbital Mech. Book). It works with all inclination ad eccentricity of s/c orbit.
  note: Subsystem1
  note: Subsystem
  S_mn : Inport
  r_mn : Inport  Port=2
  Add : Sum
  Add1 : Sum  Inputs=+-
  Constant : Constant  Value=R_t
  Constant1 : Constant
  Constant2 : Constant  Value=0
  Divide : Product  Inputs=*/
  Divide1 : Product  Inputs=*/
  Divide2 : Product  Inputs=*/
  Dot Product : DotProduct  InputSameDT=on  OutDataTypeStr=Inherit: Inherit via internal rule
  Math Function : Math  Operator=square  SaturateOnIntegerOverflow=on
  Math Function1 : Math  Operator=square  SaturateOnIntegerOverflow=on
  Product : Product
  Scope1 : Scope
  Sqrt : Sqrt  SaturateOnIntegerOverflow=on
  Sqrt1 : Sqrt  SaturateOnIntegerOverflow=on
  Sum of Elements : Sum  Inputs=+
  Sum of Elements1 : Sum  Inputs=+
  Switch : Switch
  Trigonometric Function : Trigonometry  Operator=acos
  Trigonometric Function1 : Trigonometry  Operator=acos
  Trigonometric Function2 : Trigonometry  Operator=acos
  ON/OFF : Outport
  wires:
  Switch/1 -> Scope1/1, ON/OFF/1
  Sum of Elements/1 -> Sqrt/1
  Math Function/1 -> Sum of Elements/1
  Divide1/1 -> Trigonometric Function1/1
  Math Function1/1 -> Sum of Elements1/1
  r_mn/1 -> Dot Product/2, Math Function1/1
  Dot Product/1 -> Divide/1
  Divide2/1 -> Trigonometric Function2/1
  Sqrt/1 -> Product/1, Divide1/2
  Product/1 -> Divide/2
  Sqrt1/1 -> Product/2, Divide2/2
  S_mn/1 -> Math Function/1, Dot Product/1
  Constant/1 -> Divide1/1, Divide2/1
  Sum of Elements1/1 -> Sqrt1/1
  Divide/1 -> Trigonometric Function/1
  Trigonometric Function/1 -> Add1/2
  Trigonometric Function2/1 -> Add/2
  Trigonometric Function1/1 -> Add/1
  Constant2/1 -> Switch/3
  Constant1/1 -> Switch/1
  Add1/1 -> Switch/2
  Add/1 -> Add1/1

== system saturn_thermal5/Subsystem/Eclipses System1/Saturn-Titan-SC/S//C-Titan orbit/Inertial Orbit Direction (Theta) ==
  note: definition of orbital path:
      |
      | cos(theta(t)) position wrt X_inertial (Gamma line for example)
      |
      | sin(theta(t))*cos(i) position wrt the Y_inertial
      |
      | sin(theta(t))*sin(i) position wrt the Z-inertial
      |
      | This vector define the s/c postition around the earth
  Theta : Inport
  Constant : Constant  Value=incl_sc
  Mux : Mux  Inputs=3
  Product : Product
  Product1 : Product
  Scope : Scope
  Trigonometric Function : Trigonometry
  Trigonometric Function1 : Trigonometry  Operator=cos
  Trigonometric Function2 : Trigonometry
  Trigonometric Function3 : Trigonometry  Operator=cos
  Trigonometric Function4 : Trigonometry
  r_vn : Outport
  wires:
  Product/1 -> Mux/2
  Product1/1 -> Mux/3
  Theta/1 -> Trigonometric Function1/1, Trigonometric Function/1, Trigonometric Function2/1
  Constant/1 -> Trigonometric Function3/1, Trigonometric Function4/1
  Trigonometric Function/1 -> Product/1
  Trigonometric Function1/1 -> Mux/1
  Trigonometric Function3/1 -> Product/2
  Trigonometric Function2/1 -> Product1/1
  Trigonometric Function4/1 -> Product1/2
  Mux/1 -> Scope/1, r_vn/1

== system saturn_thermal5/Subsystem/Eclipses System1/Saturn-Titan-SC/S//C-Titan orbit/Inertial Orbit Radius(Theta) ==
  note: Orbital Radius magnitude computed as function of theta:
      |
      | R= a(1-ecc^2)/(1+ ecc*cos(theta(t))
  Theta : Inport
  Add : Sum
  Constant10 : Constant  Value=ecc_sc
  Constant3 : Constant  Value=semajax_sc
  Constant5 : Constant  Value=(1 - ecc_sc^2)
  Constant9 : Constant
  Divide1 : Product  Inputs=*/
  Product : Product
  Product1 : Product
  Trigonometric Function1 : Trigonometry  Operator=cos
  r_mn : Outport
  wires:
  Product1/1 -> Add/2
  Add/1 -> Divide1/2
  Divide1/1 -> r_mn/1
  Constant9/1 -> Add/1
  Trigonometric Function1/1 -> Product1/2
  Constant5/1 -> Product/2
  Product/1 -> Divide1/1
  Theta/1 -> Trigonometric Function1/1
  Constant10/1 -> Product1/1
  Constant3/1 -> Product/1

== system saturn_thermal5/Subsystem/Eclipses System1/Saturn-Titan-SC/S//C-Titan orbit/Subsystem ==
  r_mn : Inport
  Add : Sum  Inputs=+-
  Constant1 : Constant  Value=mu_t
  Constant2 : Constant  Value=2
  Constant4 : Constant  Value=1/semajax_sc
  Divide : Product  Inputs=**
  Divide1 : Product  Inputs=*/
  Divide2 : Product  Inputs=*/
  Scope : Scope
  Scope1 : Scope
  Square Root : Sqrt  SaturateOnIntegerOverflow=on
  wires:
  Add/1 -> Divide/2
  Constant2/1 -> Divide2/1
  Constant1/1 -> Divide/1
  Divide2/1 -> Add/1
  Constant4/1 -> Add/2
  Divide/1 -> Square Root/1
  r_mn/1 -> Divide1/2, Divide2/2
  Square Root/1 -> Divide1/1, Scope/1  "v_orb"
  Divide1/1 -> Scope1/1  "w_orb"

== system saturn_thermal5/Subsystem/Eclipses System1/Saturn-Titan-SC/S//C-Titan orbit/True anomaly integration ==
  Add1 : Sum
  Add2 : Sum  Inputs=+-
  Constant1 : Constant  Value=ecc_sc
  Constant7 : Constant
  Constant8 : Constant  Value=3/2
  Divide2 : Product  Inputs=*/
  Gain : Gain  Gain=ecc_sc
  Gain1 : Gain  Gain=mean_motion_sc
  Integrator : Integrator
  Math Function : Math  Operator=pow  SaturateOnIntegerOverflow=on
  Math Function1 : Math  Operator=square  SaturateOnIntegerOverflow=on
  Math Function2 : Math  Operator=square  SaturateOnIntegerOverflow=on
  Scope : Scope
  Trigonometric Function : Trigonometry  Operator=cos
  Theta : Outport
  wires:
  Gain/1 -> Add1/1
  Constant7/1 -> Add1/2, Add2/1
  Integrator/1 -> Trigonometric Function/1, Scope/1, Theta/1  "Theta"
  Divide2/1 -> Integrator/1  "Theta_dot"
  Add1/1 -> Math Function1/1
  Math Function/1 -> Divide2/2
  Trigonometric Function/1 -> Gain/1
  Gain1/1 -> Divide2/1
  Constant8/1 -> Math Function/2
  Math Function1/1 -> Gain1/1
  Constant1/1 -> Math Function2/1
  Math Function2/1 -> Add2/2
  Add2/1 -> Math Function/1

== system saturn_thermal5/Subsystem/Eclipses System1/Saturn-Titan-SC/Titan-Saturn orbit/Subsystem ==
  note: Note: if the sun direction and the earth direction are parallel the Attitude Determinantion Algorithm wil stop to work due to sigularity value in the inertial frame direction (this matrix need to be invertible) so the theta sun integration must start with a value different from 0 or 180 deg. The alignament condition will arise again after a certain number of orbit periods (in 4 orbits this condition will not arise).
  Constant2 : Constant  Value=2*pi
  Constant3 : Constant  Value=period_t
  Divide : Product  Inputs=*/
  Integrator : Integrator
  Scope : Scope
  theta_titan : Outport
  wires:
  Constant2/1 -> Divide/1
  Constant3/1 -> Divide/2
  Divide/1 -> Integrator/1  "n_sun"
  Integrator/1 -> theta_titan/1, Scope/1

== system saturn_thermal5/Subsystem/Eclipses System1/Sun-Saturn-Titan/Saturn-Sun orbit/Subsystem ==
  Constant2 : Constant  Value=2*pi
  Constant3 : Constant  Value=period_s
  Divide : Product  Inputs=*/
  Integrator : Integrator  InitialCondition=pi/2
  Scope : Scope
  theta_saturn : Outport
  wires:
  Integrator/1 -> Scope/1, theta_saturn/1
  Divide/1 -> Integrator/1  "n_saturn"
  Constant3/1 -> Divide/2
  Constant2/1 -> Divide/1

== system saturn_thermal5/Subsystem/Eclipses System1/Sun-Saturn-Titan/Titan-Saturn/Inertial Orbit Direction (Theta) ==
  note: definition of orbital path:
      |
      | cos(theta(t)) position wrt X_inertial (Gamma line for example)
      |
      | sin(theta(t))*cos(i) position wrt the Y_inertial
      |
      | sin(theta(t))*sin(i) position wrt the Z-inertial
      |
      | This vector define the s/c postition around the earth
  Theta : Inport
  Constant : Constant  Value=incl_t
  Mux : Mux  Inputs=3
  Product : Product
  Product1 : Product
  Scope : Scope
  Trigonometric Function : Trigonometry
  Trigonometric Function1 : Trigonometry  Operator=cos
  Trigonometric Function2 : Trigonometry
  Trigonometric Function3 : Trigonometry  Operator=cos
  Trigonometric Function4 : Trigonometry
  r_vn : Outport
  wires:
  Mux/1 -> r_vn/1, Scope/1
  Trigonometric Function4/1 -> Product1/2
  Trigonometric Function2/1 -> Product1/1
  Trigonometric Function3/1 -> Product/2
  Trigonometric Function1/1 -> Mux/1
  Trigonometric Function/1 -> Product/1
  Constant/1 -> Trigonometric Function4/1, Trigonometric Function3/1
  Theta/1 -> Trigonometric Function2/1, Trigonometric Function/1, Trigonometric Function1/1
  Product1/1 -> Mux/3
  Product/1 -> Mux/2

== system saturn_thermal5/Subsystem/Eclipses System1/Sun-Saturn-Titan/Titan-Saturn/Inertial Orbit Radius(Theta) ==
  note: Orbital Radius magnitude computed as function of theta:
      |
      | R= a(1-ecc^2)/(1+ ecc*cos(theta(t))
  Theta : Inport
  Add : Sum
  Constant10 : Constant  Value=ecc_t
  Constant3 : Constant  Value=semajax_t
  Constant5 : Constant  Value=(1 - ecc_t^2)
  Constant9 : Constant
  Divide1 : Product  Inputs=*/
  Product : Product
  Product1 : Product
  Trigonometric Function1 : Trigonometry  Operator=cos
  r_mn : Outport
  wires:
  Constant3/1 -> Product/1
  Constant10/1 -> Product1/1
  Theta/1 -> Trigonometric Function1/1
  Product/1 -> Divide1/1
  Constant5/1 -> Product/2
  Trigonometric Function1/1 -> Product1/2
  Constant9/1 -> Add/1
  Divide1/1 -> r_mn/1
  Add/1 -> Divide1/2
  Product1/1 -> Add/2

== system saturn_thermal5/Subsystem/Eclipses System1/Sun-Saturn-Titan/Titan-Saturn/Subsystem ==
  r_mn : Inport
  Add : Sum  Inputs=+-
  Constant1 : Constant  Value=mu_s
  Constant2 : Constant  Value=2
  Constant4 : Constant  Value=1/semajax_t
  Divide : Product  Inputs=**
  Divide1 : Product  Inputs=*/
  Divide2 : Product  Inputs=*/
  Scope : Scope
  Scope1 : Scope
  Square Root : Sqrt  SaturateOnIntegerOverflow=on
  wires:
  Divide1/1 -> Scope1/1  "w_orb"
  Square Root/1 -> Scope/1, Divide1/1  "v_orb"
  r_mn/1 -> Divide2/2, Divide1/2
  Divide/1 -> Square Root/1
  Constant4/1 -> Add/2
  Divide2/1 -> Add/1
  Constant1/1 -> Divide/1
  Constant2/1 -> Divide2/1
  Add/1 -> Divide/2

== system saturn_thermal5/Subsystem/Eclipses System1/Sun-Saturn-Titan/Titan-Saturn/True anomaly integration ==
  Add1 : Sum
  Add2 : Sum  Inputs=+-
  Constant1 : Constant  Value=ecc_t
  Constant7 : Constant
  Constant8 : Constant  Value=3/2
  Divide2 : Product  Inputs=*/
  Gain : Gain  Gain=ecc_t
  Gain1 : Gain  Gain=mean_motion_t
  Integrator : Integrator
  Math Function : Math  Operator=pow  SaturateOnIntegerOverflow=on
  Math Function1 : Math  Operator=square  SaturateOnIntegerOverflow=on
  Math Function2 : Math  Operator=square  SaturateOnIntegerOverflow=on
  Scope : Scope
  Trigonometric Function : Trigonometry  Operator=cos
  Theta : Outport
  wires:
  Add2/1 -> Math Function/1
  Math Function2/1 -> Add2/2
  Constant1/1 -> Math Function2/1
  Math Function1/1 -> Gain1/1
  Constant8/1 -> Math Function/2
  Gain1/1 -> Divide2/1
  Trigonometric Function/1 -> Gain/1
  Math Function/1 -> Divide2/2
  Add1/1 -> Math Function1/1
  Divide2/1 -> Integrator/1  "Theta_dot"
  Integrator/1 -> Theta/1, Scope/1, Trigonometric Function/1  "Theta"
  Constant7/1 -> Add2/1, Add1/2
  Gain/1 -> Add1/1

== system saturn_thermal5/Subsystem/Eclipses System1/Sun-Titan-SC/Ecliptic Orbital parameter1/Subsystem ==
  note: Note: if the sun direction and the earth direction are parallel the Attitude Determinantion Algorithm wil stop to work due to sigularity value in the inertial frame direction (this matrix need to be invertible) so the theta sun integration must start with a value different from 0 or 180 deg. The alignament condition will arise again after a certain number of orbit periods (in 4 orbits this condition will not arise).
  Constant2 : Constant  Value=2*pi
  Constant3 : Constant  Value=period_s
  Divide : Product  Inputs=*/
  Integrator : Integrator  InitialCondition=pi/2
  Scope : Scope
  theta_sun : Outport
  wires:
  Constant2/1 -> Divide/1
  Constant3/1 -> Divide/2
  Divide/1 -> Integrator/1  "n_sun"
  Integrator/1 -> theta_sun/1, Scope/1
